simulink model "Prova_SITL_GPS"  (R2020b)
settings: Solver=VariableStepAuto  StartTime=0.0  StopTime=5  RelTol=1e-3
settings Model: Creator=User  LastModifiedBy=david

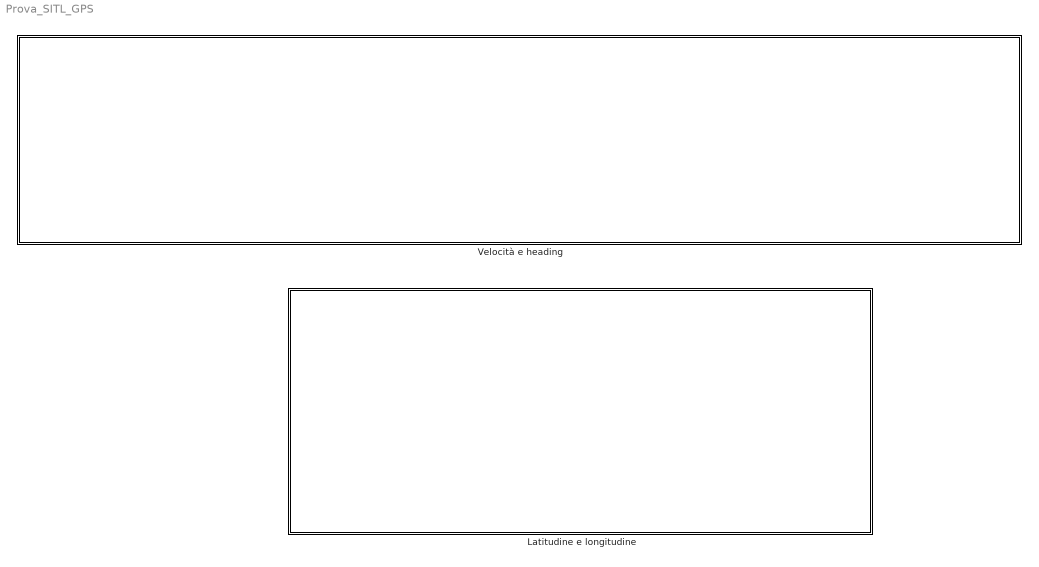
== system Prova_SITL_GPS ==
  Latitudine e longitudine : Subsystem
  Velocità e heading : Subsystem

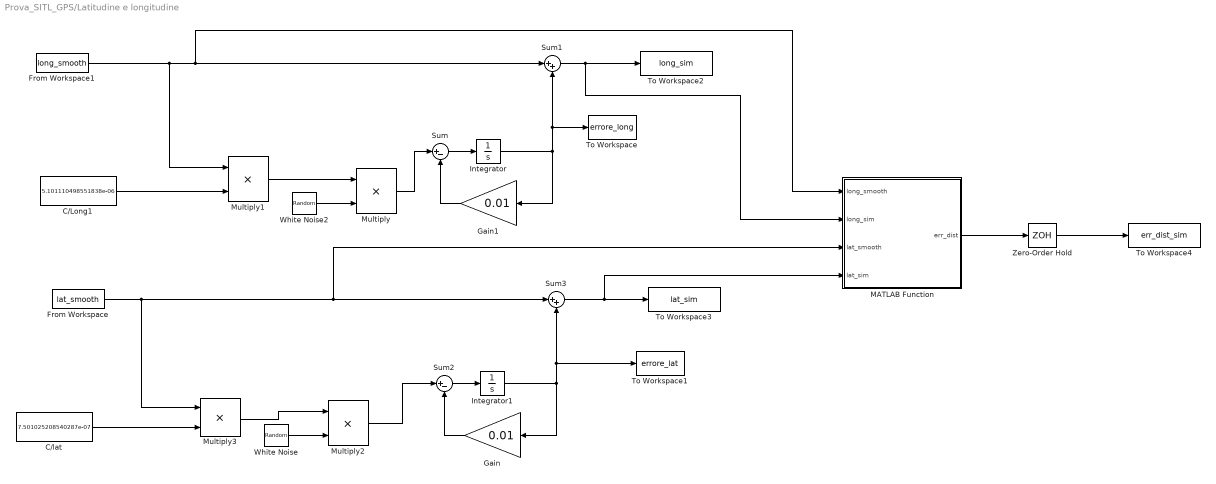
== system Prova_SITL_GPS/Latitudine e longitudine ==
  C/Long1 : Constant  Value=5.101110498551838e-06
  C/lat : Constant  Value=7.501025208540287e-07
  From Workspace : FromWorkspace  VariableName=lat_smooth
  From Workspace1 : FromWorkspace  VariableName=long_smooth
  Gain : Gain  Gain=0.01  SaturateOnIntegerOverflow=on  OutDataTypeStr=Inherit: Same as input  ParamDataTypeStr=Inherit: Same as input
  Gain1 : Gain  Gain=0.01  SaturateOnIntegerOverflow=on  OutDataTypeStr=Inherit: Same as input  ParamDataTypeStr=Inherit: Same as input
  Integrator : Integrator
  Integrator1 : Integrator
  MATLAB Function : MATLAB Function  TreatAsAtomicUnit=on
  Multiply{,1..3} (4 alike) : Product
  Sum : Sum  Inputs=|+-  InputSameDT=on  SaturateOnIntegerOverflow=on  OutDataTypeStr=Inherit: Same as first input
  Sum1 : Sum  Inputs=|++  InputSameDT=on  SaturateOnIntegerOverflow=on  OutDataTypeStr=Inherit: Same as first input
  Sum2 : Sum  Inputs=|+-  InputSameDT=on  SaturateOnIntegerOverflow=on  OutDataTypeStr=Inherit: Same as first input
  Sum3 : Sum  Inputs=|++  InputSameDT=on  SaturateOnIntegerOverflow=on  OutDataTypeStr=Inherit: Same as first input
  To Workspace : ToWorkspace  VariableName=errore_long  SampleTime=-1
      settings: Save2DSignal=2-D array (concatenate along first dimension)
  To Workspace1 : ToWorkspace  VariableName=errore_lat  SampleTime=-1
      settings: Save2DSignal=2-D array (concatenate along first dimension)
  To Workspace2 : ToWorkspace  VariableName=long_sim  SampleTime=-1
      settings: Save2DSignal=2-D array (concatenate along first dimension)
  To Workspace3 : ToWorkspace  VariableName=lat_sim  SampleTime=-1
      settings: Save2DSignal=2-D array (concatenate along first dimension)
  To Workspace4 : ToWorkspace  VariableName=err_dist_sim  SampleTime=-1
      settings: Save2DSignal=2-D array (concatenate along first dimension)
  White Noise : RandomNumber  Seed=randi([0 2000],1,1)  SampleTime=0.1
  White Noise2 : RandomNumber  Seed=randi([0 2000],1,1)  SampleTime=0.1
  Zero-Order Hold : ZeroOrderHold  SampleTime=0.02
  wires:
  Integrator/1 -> Sum1/2, To Workspace/1, Gain1/1
  Sum/1 -> Integrator/1
  Sum1/1 -> MATLAB Function/2(long_sim), To Workspace2/1
  Gain1/1 -> Sum/2
  Gain/1 -> Sum2/2
  Integrator1/1 -> Gain/1, Sum3/2, To Workspace1/1
  Sum3/1 -> MATLAB Function/4(lat_sim), To Workspace3/1
  Sum2/1 -> Integrator1/1
  MATLAB Function/1(err_dist) -> Zero-Order Hold/1
  Zero-Order Hold/1 -> To Workspace4/1
  Multiply1/1 -> Multiply/1
  Multiply/1 -> Sum/1
  C/Long1/1 -> Multiply1/2
  White Noise2/1 -> Multiply/2
  From Workspace1/1 -> Multiply1/1, MATLAB Function/1(long_smooth), Sum1/1
  Multiply3/1 -> Multiply2/1
  Multiply2/1 -> Sum2/1
  C/lat/1 -> Multiply3/2
  White Noise/1 -> Multiply2/2
  From Workspace/1 -> MATLAB Function/3(lat_smooth), Sum3/1, Multiply3/1

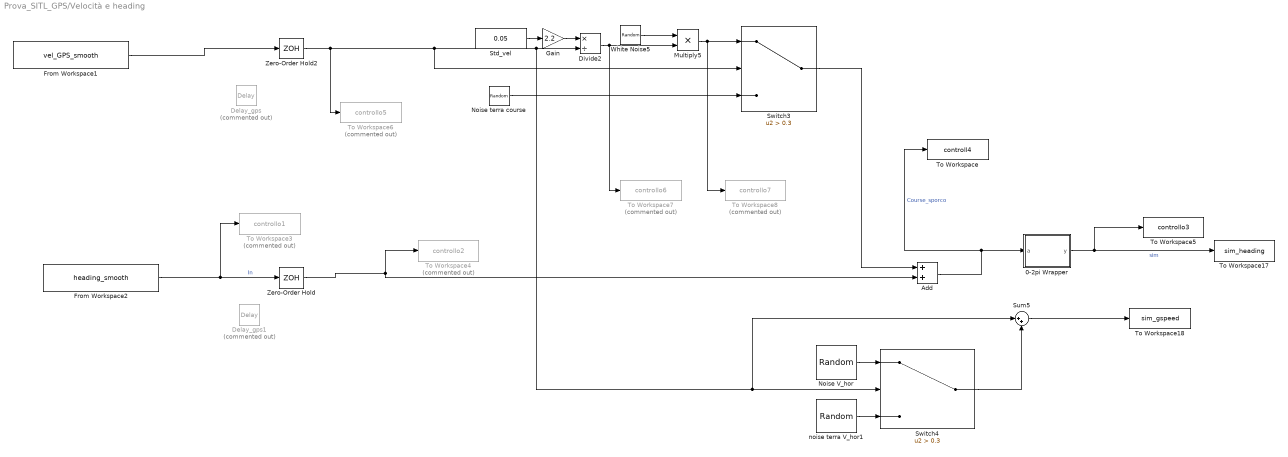
== system Prova_SITL_GPS/Velocità e heading ==
  0-2pi Wrapper : MATLAB Function  TreatAsAtomicUnit=on
  Add : Sum
  Delay_gps : TransportDelay  Commented=on  DelayTime=0
  Delay_gps1 : TransportDelay  Commented=on  DelayTime=0
  Divide2 : Product  Inputs=*/
  From Workspace1 : FromWorkspace  VariableName=vel_GPS_smooth
  From Workspace2 : FromWorkspace  VariableName=heading_smooth
  Gain : Gain  Gain=2.2
  Multiply5 : Product
  Noise V_hor : RandomNumber  Variance=0.0025  Seed=randi([0 2000],1,1)  SampleTime=0.1
  Noise terra course : RandomNumber  Variance=0.04  Seed=randi([0 2000],1,1)  SampleTime=0.1
  Std_vel : Constant  Value=0.05  SampleTime=0.1
  Sum5 : Sum  Inputs=|++
  Switch3 : Switch  Criteria=u2 > Threshold  Threshold=0.3
  Switch4 : Switch  Criteria=u2 > Threshold  Threshold=0.3
  To Workspace : ToWorkspace  VariableName=controll4  SampleTime=-1
  To Workspace17 : ToWorkspace  VariableName=sim_heading  SampleTime=-1
  To Workspace18 : ToWorkspace  VariableName=sim_gspeed  SampleTime=-1
  To Workspace3 : ToWorkspace  Commented=on  VariableName=controllo1  SampleTime=-1
      settings: Save2DSignal=2-D array (concatenate along first dimension)
  To Workspace4 : ToWorkspace  Commented=on  VariableName=controllo2  SampleTime=-1
      settings: Save2DSignal=2-D array (concatenate along first dimension)
  To Workspace5 : ToWorkspace  VariableName=controllo3  SampleTime=-1
      settings: Save2DSignal=2-D array (concatenate along first dimension)
  To Workspace6 : ToWorkspace  Commented=on  VariableName=controllo5  SampleTime=-1
      settings: Save2DSignal=2-D array (concatenate along first dimension)
  To Workspace7 : ToWorkspace  Commented=on  VariableName=controllo6  SampleTime=-1
      settings: Save2DSignal=2-D array (concatenate along first dimension)
  To Workspace8 : ToWorkspace  Commented=on  VariableName=controllo7  SampleTime=-1
      settings: Save2DSignal=2-D array (concatenate along first dimension)
  White Noise5 : RandomNumber  Variance=0.1  Seed=randi([0 2000],1,1)  SampleTime=0.1
  Zero-Order Hold : ZeroOrderHold  SampleTime=0.02
  Zero-Order Hold2 : ZeroOrderHold  SampleTime=0.02
  noise terra V_hor1 : RandomNumber  Variance=0.0625  Seed=randi([0 2000],1,1)  SampleTime=0.1
  wires:
  Gain/1 -> Divide2/1
  Noise terra course/1 -> Switch3/3
  Divide2/1 -> To Workspace7/1, Multiply5/2
  Std_vel/1 -> Gain/1
  Multiply5/1 -> Switch3/1, To Workspace8/1
  Zero-Order Hold2/1 -> To Workspace6/1, Divide2/2, Switch4/2, Sum5/1, Switch3/2
  From Workspace2/1 -> To Workspace3/1, Zero-Order Hold/1  "In"
  Zero-Order Hold/1 -> Add/2, To Workspace4/1
  Switch4/1 -> Sum5/2
  White Noise5/1 -> Multiply5/1
  0-2pi Wrapper/1(y) -> To Workspace17/1, To Workspace5/1  "sim"
  Switch3/1 -> Add/1
  Noise V_hor/1 -> Switch4/1
  From Workspace1/1 -> Zero-Order Hold2/1
  Sum5/1 -> To Workspace18/1
  noise terra V_hor1/1 -> Switch4/3
  Add/1 -> 0-2pi Wrapper/1(a), To Workspace/1  "Course_sporco"

== matlab function Prova_SITL_GPS/Latitudine e longitudine/MATLAB Function ==
  data: long_smooth input; long_sim input; lat_smooth input; err_dist output; lat_sim input
function err_dist = haversine(long_smooth,long_sim,lat_smooth,lat_sim )

r=6371*10^3; %raggio terra in m


err_dist = 2*r*asin(sqrt(sin((lat_smooth-lat_sim)/2)^2+cos(lat_sim)*cos(lat_smooth)*sin((long_smooth-long_sim)/2)^2 ));

== matlab function Prova_SITL_GPS/Velocità e heading/0-2pi Wrapper ==
  data: a input; y output
function y = fcn(a)
%% Wrapper da [-180,+180] a [0,360]
%https://stackoverflow.com/questions/11498169/dealing-with-angle-wrap-in-c-code
close all

b=2*pi;

k=floor(a/b);
fmod=a-k*b;


if fmod<0
    
   fmod=fmod+2*pi;
    
end

y=fmod;
